simulink model "BLEMeshPDRvsRateModel"  (R2021a)
settings: Solver=VariableStepDiscrete  StartTime=0.0  StopTime=5  MaxStep=inf  RelTol=1e-3
PostLoadFcn:
  | load('bleMeshBusObjects.mat');
  | load('bleMeshDESNodePositions.mat');
  | ModelName = bdroot;
  | helperBLEMeshAssignNodeIDs(ModelName);
  | NumberOfNodes = numel(helperBLEMeshGetNodeNamesList(ModelName));
  | % Statistics
  | opcode = 0; % For creating the table
  | helperBLEMeshUpdateStatistics(opcode);
  | meshNetworkGraph = helperBLEMeshVisualizeNetwork();
InitFcn:
  | load('bleMeshBusObjects.mat');
  | load('bleMeshDESNodePositions.mat');
  | ModelName = bdroot;
  | helperBLEMeshAssignNodeIDs(ModelName);
  | NumberOfNodes = numel(helperBLEMeshGetNodeNamesList(ModelName));
  | % Statistics
  | opcode = 0; % For creating the table
  | helperBLEMeshUpdateStatistics(opcode);
  | meshNetworkGraph = helperBLEMeshVisualizeNetwork();
  | rng('default');
StartFcn:
  | if enableVisualization == 1
  | meshNetworkGraph.createNetwork();
  | end
StopFcn:
  | % Sort statisticsAtEachNode table
  | list = statisticsAtEachNode.Properties.RowNames;
  | nodeNum = cellfun(@(x)sscanf(x,'Node%d'), list);
  | [~,sortIdx] = sort(nodeNum);
  | statisticsAtEachNode = statisticsAtEachNode(sortIdx, :);
  | 
  | % Fill node statisticsAtEachNode in a cell array as input to visualization object
  | nodeStatistics = cell(1, NumberOfNodes);
  | for idx = 1:NumberOfNodes
  |     stats = {
  |         'Node Type', statisticsAtEachNode{idx, 'NodeType'}, ...
  |         'PHYTransmittedSignals', statisticsAtEachNode{idx, 'PHYTransmittedSignals'}, ...
  |         'PHYReceivedSignals', statisticsAtEachNode{idx, 'PHYReceivedSignals'}, ...
  |         'TotalCollisions', statisticsAtEachNode{idx, 'TotalCollisions'}, ...
  |         'LinkLayerTransmittedMsgs', statisticsAtEachNode{idx, 'LinkLayerTransmittedMsgs'}, ...
  |         'LinkLayerReceivedMsgs', statisticsAtEachNode{idx, 'LinkLayerReceivedMsgs'}, ...
  |         'CRCFailedMsgs', statisticsAtEachNode{idx, 'CRCFailedMsgs'}, ...
  |         'NetworkLayerTransmittedMsgs', statisticsAtEachNode{idx, 'NetworkLayerTransmittedMsgs'}, ...
  |         'NetworkLayerReceivedMsgs', statisticsAtEachNode{idx, 'NetworkLayerReceivedMsgs'}, ...
  |         'ReceivedApplicationMsgs', statisticsAtEachNode{idx, 'ReceivedApplicationMsgs'}, ...
  |         'NetworkLayerRelayedMsgs', statisticsAtEachNode{idx, 'NetworkLayerRelayedMsgs'}, ...
  |         'NetworkLayerDroppedMsgs', statisticsAtEachNode{idx, 'NetworkLayerDroppedMsgs'}};
  |     nodeStatistics{idx} = stats;
  | end
  | % Update statisticsAtEachNode in visualization object
  | if enableVisualization == 1
  | meshNetworkGraph.updateNodeStatistics(nodeStatistics);
  | end
  | % Calculate PDR of network
  | PDR = sum(statisticsAtEachNode.ReceivedApplicationMsgs) / sum(statisticsAtEachNode.NetworkLayerTransmittedMsgs);
  | fprintf('Network PDR is: %f\n', round(PDR, 4));
values from neighbouring files (symbols this model uses):
  bleMeshDESNodePositions = [0 2 4 6 8 10 12 14 16 18 20 22 ... (300 elements, 100x3)]    [bleMeshDESNodePositions.mat]    (also in bleMeshDESNodePositions19.mat = [5.030833333 8.024583333 13.395 16.32708333 22.90125 22.9012; bleMeshDESNodePositions38.mat = [2.7 5.45 5.825 10.65 13.5 13.875 18.65 21.4 18.55 2.7 5.45 ; bleMeshDESNodePositions51.mat = [2.45 5.4 2.45 5.4 5.75 10.375 13.3 10.375 13.3 13.75 18.75 ; bleMeshDESNodePositions68.mat = [0 2 4 6 8 10 12 14 16 18 0 2 ... (300 elements, 100x3)])
undefined symbols (not defined in the file or in its folder): m
libraries: BLEMeshLib x260
(part 2 of 5)

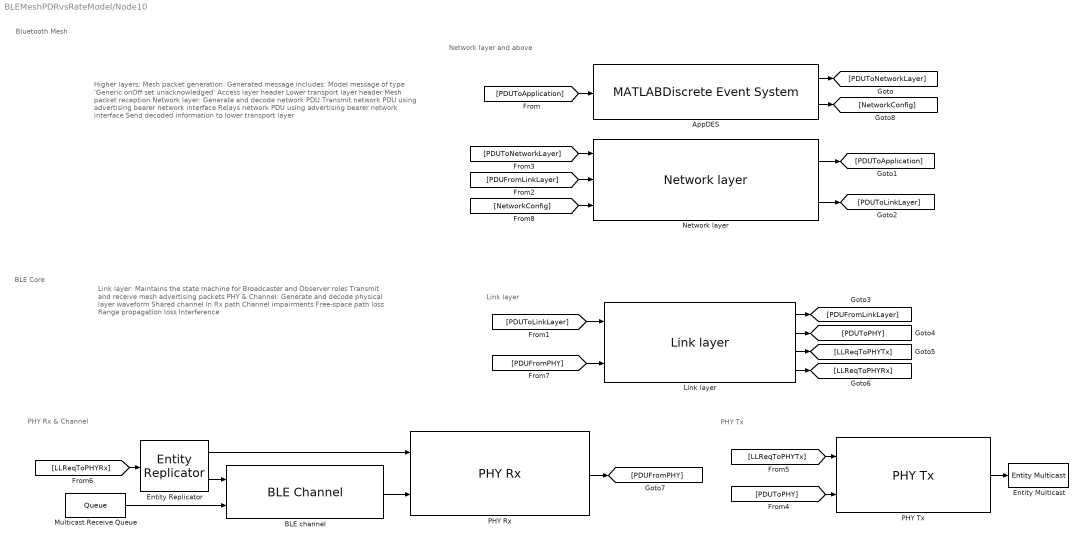
== system BLEMeshPDRvsRateModel/Node10 ==
  note: Network layer and above
  note: Link layer
  note: Link layer:
      | Maintains the state machine for Broadcaster and Observer roles
      | Transmit and receive mesh advertising packets
      |
      | PHY & Channel:
      | Generate and decode physical layer waveform
      | Shared channel in Rx path
      | Channel impairments
      | Free-space path loss
      | Range propagation loss
      | Interference
  note: BLE Core
  note: Bluetooth Mesh
  note: PHY Rx & Channel
  note: PHY Tx
  note: Higher layers:
      | Mesh packet generation. Generated message includes:
      | Model message of type 'Generic onOff set unacknowledged'
      | Access layer header
      | Lower transport layer header
      | Mesh packet reception
      |
      | Network layer:
      | Generate and decode network PDU
      | Transmit network PDU using advertising bearer network interface
      | Relays network PDU using advertising bearer network interface
      | Send decoded information to lower transport layer
  AppDES : MATLABDiscreteEventSystem  InputPortMessageModes=m  OutputPortMessageModes=m,m  System=AppDES  NodeID=1  DestinationNode=1  ApplicationState=0  TTL=127  SourceRate=1  TotalPackets=1  SimulateUsing=Code generation
      mask Type: AppDES
      mask Display:
      | disp('AppDES');
      | port_label('input',1,'transportPDUIn');
      | port_label('output',1,'transportPDUOut');
      | port_label('output',2,'networkConfig');
  BLE channel : BLEMeshLib/BLE Channel  RangePropagationLoss=On  FSPLModel=On  RxRange=8  NodePosition=NodePosition  NodeID=NodeID  SimulateUsing=Code generation
  Entity Multicast : EntityMulticast  InputPortMessageModes=m  MulticastTag=channel
  Entity Replicator : EntityReplicator  InputPortMessageModes=m  OutputPortMessageModes=m,m
  Link layer : BLEMeshLib/Link layer  RandomAdvertising=On  AdvertisingInterval=20  ScanInterval=30  NodeID=NodeID  SimulateUsing=Code generation  mask(helperBLEMeshLinkLayerDES){}
  Multicast Receive Queue : Queue  OutputPortMessageModes=m  EntityArrivalSource=Multicast  MulticastTag=channel
  Network layer : BLEMeshLib/Network layer  Relay=Off  ElementAddresses=ElementAddress  NetworkTransmitCount=3  NetworkTransmitInterval=30  RelayRetransmitCount=3  RelayRetransmitInterval=30  NodeID=NodeID  SimulateUsing=Code generation
  PHY Rx : BLEMeshLib/PHY Rx  NoiseFigure=0  NodeID=NodeID  SimulateUsing=Interpreted execution
  PHY Tx : BLEMeshLib/PHY Tx  TxPower=0  NodePosition=NodePosition  NodeID=NodeID  SimulateUsing=Interpreted execution
  wires:
  Link layer/4 -> [LLReqToPHYRx]
  Link layer/2 -> [PDUToPHY]
  Link layer/3 -> [LLReqToPHYTx]
  Link layer/1 -> [PDUFromLinkLayer]
  [PDUToNetworkLayer] -> Network layer/1
  Network layer/1 -> [PDUToApplication]
  [PDUFromLinkLayer] -> Network layer/2
  Entity Replicator/1 -> PHY Rx/1
  PHY Rx/1 -> [PDUFromPHY]
  BLE channel/1 -> PHY Rx/2
  PHY Tx/1 -> Entity Multicast/1
  [LLReqToPHYRx] -> Entity Replicator/1
  Multicast Receive Queue/1 -> BLE channel/2
  Entity Replicator/2 -> BLE channel/1
  [LLReqToPHYTx] -> PHY Tx/1
  [PDUToPHY] -> PHY Tx/2
  Network layer/2 -> [PDUToLinkLayer]
  [PDUToLinkLayer] -> Link layer/1
  [PDUFromPHY] -> Link layer/2
  AppDES/1 -> [PDUToNetworkLayer]
  [PDUToApplication] -> AppDES/1
  [NetworkConfig] -> Network layer/3
  AppDES/2 -> [NetworkConfig]

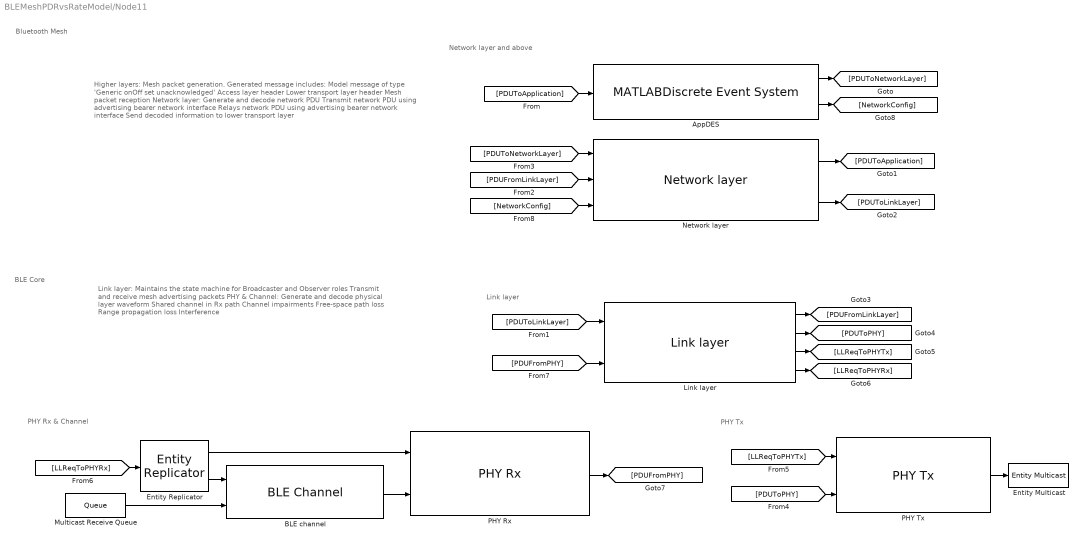
== system BLEMeshPDRvsRateModel/Node11 ==
  note: Network layer and above
  note: Link layer
  note: Link layer:
      | Maintains the state machine for Broadcaster and Observer roles
      | Transmit and receive mesh advertising packets
      |
      | PHY & Channel:
      | Generate and decode physical layer waveform
      | Shared channel in Rx path
      | Channel impairments
      | Free-space path loss
      | Range propagation loss
      | Interference
  note: BLE Core
  note: Bluetooth Mesh
  note: PHY Rx & Channel
  note: PHY Tx
  note: Higher layers:
      | Mesh packet generation. Generated message includes:
      | Model message of type 'Generic onOff set unacknowledged'
      | Access layer header
      | Lower transport layer header
      | Mesh packet reception
      |
      | Network layer:
      | Generate and decode network PDU
      | Transmit network PDU using advertising bearer network interface
      | Relays network PDU using advertising bearer network interface
      | Send decoded information to lower transport layer
  AppDES : MATLABDiscreteEventSystem  InputPortMessageModes=m  OutputPortMessageModes=m,m  System=AppDES  NodeID=1  DestinationNode=1  ApplicationState=0  TTL=127  SourceRate=1  TotalPackets=1  SimulateUsing=Code generation
      mask Type: AppDES
      mask Display:
      | disp('AppDES');
      | port_label('input',1,'transportPDUIn');
      | port_label('output',1,'transportPDUOut');
      | port_label('output',2,'networkConfig');
  BLE channel : BLEMeshLib/BLE Channel  RangePropagationLoss=On  FSPLModel=On  RxRange=8  NodePosition=NodePosition  NodeID=NodeID  SimulateUsing=Code generation
  Entity Multicast : EntityMulticast  InputPortMessageModes=m  MulticastTag=channel
  Entity Replicator : EntityReplicator  InputPortMessageModes=m  OutputPortMessageModes=m,m
  Link layer : BLEMeshLib/Link layer  RandomAdvertising=On  AdvertisingInterval=20  ScanInterval=30  NodeID=NodeID  SimulateUsing=Code generation  mask(helperBLEMeshLinkLayerDES){}
  Multicast Receive Queue : Queue  OutputPortMessageModes=m  EntityArrivalSource=Multicast  MulticastTag=channel
  Network layer : BLEMeshLib/Network layer  Relay=On  ElementAddresses=ElementAddress  NetworkTransmitCount=3  NetworkTransmitInterval=30  RelayRetransmitCount=3  RelayRetransmitInterval=30  NodeID=NodeID  SimulateUsing=Code generation
  PHY Rx : BLEMeshLib/PHY Rx  NoiseFigure=0  NodeID=NodeID  SimulateUsing=Interpreted execution
  PHY Tx : BLEMeshLib/PHY Tx  TxPower=0  NodePosition=NodePosition  NodeID=NodeID  SimulateUsing=Interpreted execution
  wires:
  Link layer/4 -> [LLReqToPHYRx]
  Link layer/2 -> [PDUToPHY]
  Link layer/3 -> [LLReqToPHYTx]
  Link layer/1 -> [PDUFromLinkLayer]
  [PDUToNetworkLayer] -> Network layer/1
  Network layer/1 -> [PDUToApplication]
  [PDUFromLinkLayer] -> Network layer/2
  Entity Replicator/1 -> PHY Rx/1
  PHY Rx/1 -> [PDUFromPHY]
  BLE channel/1 -> PHY Rx/2
  PHY Tx/1 -> Entity Multicast/1
  [LLReqToPHYRx] -> Entity Replicator/1
  Multicast Receive Queue/1 -> BLE channel/2
  Entity Replicator/2 -> BLE channel/1
  [LLReqToPHYTx] -> PHY Tx/1
  [PDUToPHY] -> PHY Tx/2
  Network layer/2 -> [PDUToLinkLayer]
  [PDUToLinkLayer] -> Link layer/1
  [PDUFromPHY] -> Link layer/2
  AppDES/1 -> [PDUToNetworkLayer]
  [PDUToApplication] -> AppDES/1
  [NetworkConfig] -> Network layer/3
  AppDES/2 -> [NetworkConfig]

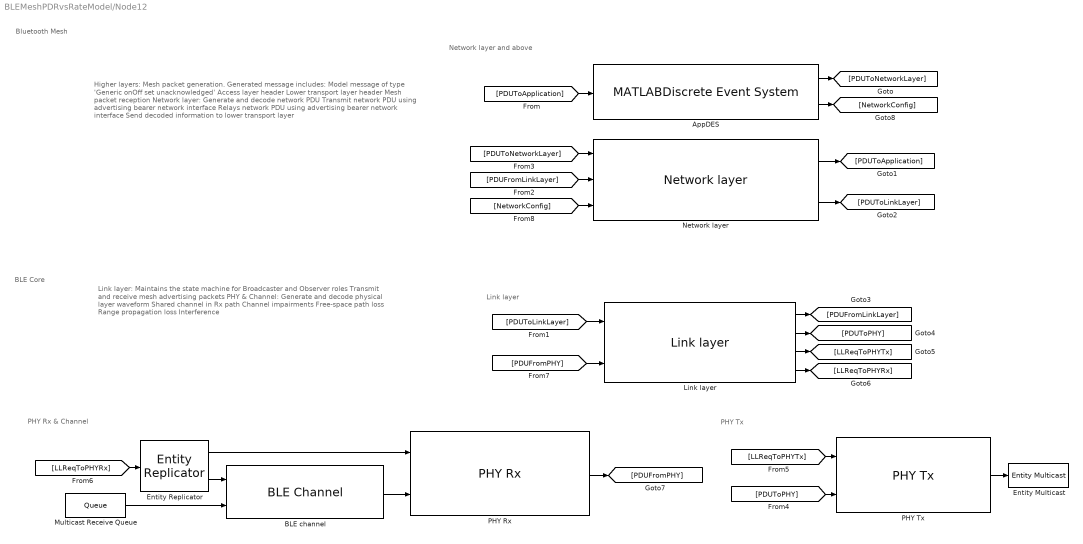
== system BLEMeshPDRvsRateModel/Node12 ==
  note: Network layer and above
  note: Link layer
  note: Link layer:
      | Maintains the state machine for Broadcaster and Observer roles
      | Transmit and receive mesh advertising packets
      |
      | PHY & Channel:
      | Generate and decode physical layer waveform
      | Shared channel in Rx path
      | Channel impairments
      | Free-space path loss
      | Range propagation loss
      | Interference
  note: BLE Core
  note: Bluetooth Mesh
  note: PHY Rx & Channel
  note: PHY Tx
  note: Higher layers:
      | Mesh packet generation. Generated message includes:
      | Model message of type 'Generic onOff set unacknowledged'
      | Access layer header
      | Lower transport layer header
      | Mesh packet reception
      |
      | Network layer:
      | Generate and decode network PDU
      | Transmit network PDU using advertising bearer network interface
      | Relays network PDU using advertising bearer network interface
      | Send decoded information to lower transport layer
  AppDES : MATLABDiscreteEventSystem  InputPortMessageModes=m  OutputPortMessageModes=m,m  System=AppDES  NodeID=1  DestinationNode=1  ApplicationState=0  TTL=127  SourceRate=1  TotalPackets=1  SimulateUsing=Code generation
      mask Type: AppDES
      mask Display:
      | disp('AppDES');
      | port_label('input',1,'transportPDUIn');
      | port_label('output',1,'transportPDUOut');
      | port_label('output',2,'networkConfig');
  BLE channel : BLEMeshLib/BLE Channel  RangePropagationLoss=On  FSPLModel=On  RxRange=8  NodePosition=NodePosition  NodeID=NodeID  SimulateUsing=Code generation
  Entity Multicast : EntityMulticast  InputPortMessageModes=m  MulticastTag=channel
  Entity Replicator : EntityReplicator  InputPortMessageModes=m  OutputPortMessageModes=m,m
  Link layer : BLEMeshLib/Link layer  RandomAdvertising=On  AdvertisingInterval=20  ScanInterval=30  NodeID=NodeID  SimulateUsing=Code generation  mask(helperBLEMeshLinkLayerDES){}
  Multicast Receive Queue : Queue  OutputPortMessageModes=m  EntityArrivalSource=Multicast  MulticastTag=channel
  Network layer : BLEMeshLib/Network layer  Relay=On  ElementAddresses=ElementAddress  NetworkTransmitCount=3  NetworkTransmitInterval=30  RelayRetransmitCount=3  RelayRetransmitInterval=30  NodeID=NodeID  SimulateUsing=Code generation
  PHY Rx : BLEMeshLib/PHY Rx  NoiseFigure=0  NodeID=NodeID  SimulateUsing=Interpreted execution
  PHY Tx : BLEMeshLib/PHY Tx  TxPower=0  NodePosition=NodePosition  NodeID=NodeID  SimulateUsing=Interpreted execution
  wires:
  Link layer/4 -> [LLReqToPHYRx]
  Link layer/2 -> [PDUToPHY]
  Link layer/3 -> [LLReqToPHYTx]
  Link layer/1 -> [PDUFromLinkLayer]
  [PDUToNetworkLayer] -> Network layer/1
  Network layer/1 -> [PDUToApplication]
  [PDUFromLinkLayer] -> Network layer/2
  Entity Replicator/1 -> PHY Rx/1
  PHY Rx/1 -> [PDUFromPHY]
  BLE channel/1 -> PHY Rx/2
  PHY Tx/1 -> Entity Multicast/1
  [LLReqToPHYRx] -> Entity Replicator/1
  Multicast Receive Queue/1 -> BLE channel/2
  Entity Replicator/2 -> BLE channel/1
  [LLReqToPHYTx] -> PHY Tx/1
  [PDUToPHY] -> PHY Tx/2
  Network layer/2 -> [PDUToLinkLayer]
  [PDUToLinkLayer] -> Link layer/1
  [PDUFromPHY] -> Link layer/2
  AppDES/1 -> [PDUToNetworkLayer]
  [PDUToApplication] -> AppDES/1
  [NetworkConfig] -> Network layer/3
  AppDES/2 -> [NetworkConfig]

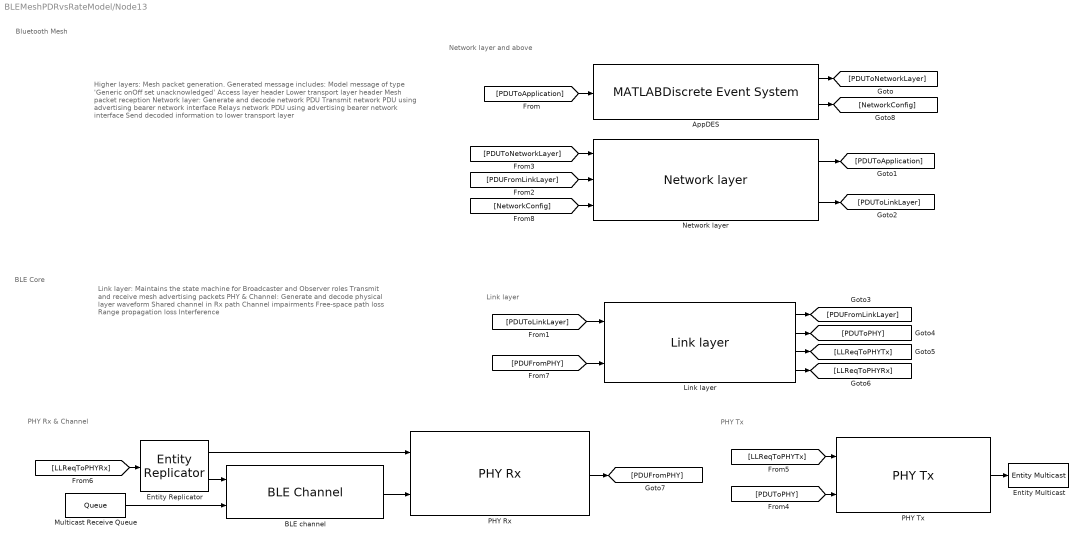
== system BLEMeshPDRvsRateModel/Node13 ==
  note: Network layer and above
  note: Link layer
  note: Link layer:
      | Maintains the state machine for Broadcaster and Observer roles
      | Transmit and receive mesh advertising packets
      |
      | PHY & Channel:
      | Generate and decode physical layer waveform
      | Shared channel in Rx path
      | Channel impairments
      | Free-space path loss
      | Range propagation loss
      | Interference
  note: BLE Core
  note: Bluetooth Mesh
  note: PHY Rx & Channel
  note: PHY Tx
  note: Higher layers:
      | Mesh packet generation. Generated message includes:
      | Model message of type 'Generic onOff set unacknowledged'
      | Access layer header
      | Lower transport layer header
      | Mesh packet reception
      |
      | Network layer:
      | Generate and decode network PDU
      | Transmit network PDU using advertising bearer network interface
      | Relays network PDU using advertising bearer network interface
      | Send decoded information to lower transport layer
  AppDES : MATLABDiscreteEventSystem  InputPortMessageModes=m  OutputPortMessageModes=m,m  System=AppDES  NodeID=1  DestinationNode=1  ApplicationState=0  TTL=127  SourceRate=1  TotalPackets=1  SimulateUsing=Code generation
      mask Type: AppDES
      mask Display:
      | disp('AppDES');
      | port_label('input',1,'transportPDUIn');
      | port_label('output',1,'transportPDUOut');
      | port_label('output',2,'networkConfig');
  BLE channel : BLEMeshLib/BLE Channel  RangePropagationLoss=On  FSPLModel=On  RxRange=8  NodePosition=NodePosition  NodeID=NodeID  SimulateUsing=Code generation
  Entity Multicast : EntityMulticast  InputPortMessageModes=m  MulticastTag=channel
  Entity Replicator : EntityReplicator  InputPortMessageModes=m  OutputPortMessageModes=m,m
  Link layer : BLEMeshLib/Link layer  RandomAdvertising=On  AdvertisingInterval=20  ScanInterval=30  NodeID=NodeID  SimulateUsing=Code generation  mask(helperBLEMeshLinkLayerDES){}
  Multicast Receive Queue : Queue  OutputPortMessageModes=m  EntityArrivalSource=Multicast  MulticastTag=channel
  Network layer : BLEMeshLib/Network layer  Relay=On  ElementAddresses=ElementAddress  NetworkTransmitCount=3  NetworkTransmitInterval=30  RelayRetransmitCount=3  RelayRetransmitInterval=30  NodeID=NodeID  SimulateUsing=Code generation
  PHY Rx : BLEMeshLib/PHY Rx  NoiseFigure=0  NodeID=NodeID  SimulateUsing=Interpreted execution
  PHY Tx : BLEMeshLib/PHY Tx  TxPower=0  NodePosition=NodePosition  NodeID=NodeID  SimulateUsing=Interpreted execution
  wires:
  Link layer/4 -> [LLReqToPHYRx]
  Link layer/2 -> [PDUToPHY]
  Link layer/3 -> [LLReqToPHYTx]
  Link layer/1 -> [PDUFromLinkLayer]
  [PDUToNetworkLayer] -> Network layer/1
  Network layer/1 -> [PDUToApplication]
  [PDUFromLinkLayer] -> Network layer/2
  Entity Replicator/1 -> PHY Rx/1
  PHY Rx/1 -> [PDUFromPHY]
  BLE channel/1 -> PHY Rx/2
  PHY Tx/1 -> Entity Multicast/1
  [LLReqToPHYRx] -> Entity Replicator/1
  Multicast Receive Queue/1 -> BLE channel/2
  Entity Replicator/2 -> BLE channel/1
  [LLReqToPHYTx] -> PHY Tx/1
  [PDUToPHY] -> PHY Tx/2
  Network layer/2 -> [PDUToLinkLayer]
  [PDUToLinkLayer] -> Link layer/1
  [PDUFromPHY] -> Link layer/2
  AppDES/1 -> [PDUToNetworkLayer]
  [PDUToApplication] -> AppDES/1
  [NetworkConfig] -> Network layer/3
  AppDES/2 -> [NetworkConfig]

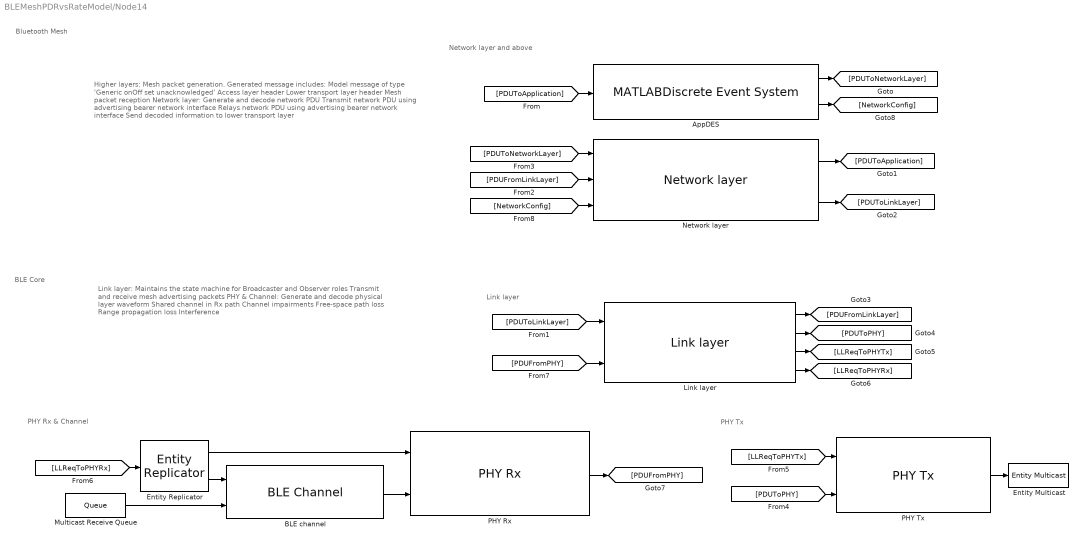
== system BLEMeshPDRvsRateModel/Node14 ==
  note: Network layer and above
  note: Link layer
  note: Link layer:
      | Maintains the state machine for Broadcaster and Observer roles
      | Transmit and receive mesh advertising packets
      |
      | PHY & Channel:
      | Generate and decode physical layer waveform
      | Shared channel in Rx path
      | Channel impairments
      | Free-space path loss
      | Range propagation loss
      | Interference
  note: BLE Core
  note: Bluetooth Mesh
  note: PHY Rx & Channel
  note: PHY Tx
  note: Higher layers:
      | Mesh packet generation. Generated message includes:
      | Model message of type 'Generic onOff set unacknowledged'
      | Access layer header
      | Lower transport layer header
      | Mesh packet reception
      |
      | Network layer:
      | Generate and decode network PDU
      | Transmit network PDU using advertising bearer network interface
      | Relays network PDU using advertising bearer network interface
      | Send decoded information to lower transport layer
  AppDES : MATLABDiscreteEventSystem  InputPortMessageModes=m  OutputPortMessageModes=m,m  System=AppDES  NodeID=1  DestinationNode=1  ApplicationState=0  TTL=127  SourceRate=1  TotalPackets=1  SimulateUsing=Code generation
      mask Type: AppDES
      mask Display:
      | disp('AppDES');
      | port_label('input',1,'transportPDUIn');
      | port_label('output',1,'transportPDUOut');
      | port_label('output',2,'networkConfig');
  BLE channel : BLEMeshLib/BLE Channel  RangePropagationLoss=On  FSPLModel=On  RxRange=8  NodePosition=NodePosition  NodeID=NodeID  SimulateUsing=Code generation
  Entity Multicast : EntityMulticast  InputPortMessageModes=m  MulticastTag=channel
  Entity Replicator : EntityReplicator  InputPortMessageModes=m  OutputPortMessageModes=m,m
  Link layer : BLEMeshLib/Link layer  RandomAdvertising=On  AdvertisingInterval=20  ScanInterval=30  NodeID=NodeID  SimulateUsing=Code generation  mask(helperBLEMeshLinkLayerDES){}
  Multicast Receive Queue : Queue  OutputPortMessageModes=m  EntityArrivalSource=Multicast  MulticastTag=channel
  Network layer : BLEMeshLib/Network layer  Relay=On  ElementAddresses=ElementAddress  NetworkTransmitCount=3  NetworkTransmitInterval=30  RelayRetransmitCount=3  RelayRetransmitInterval=30  NodeID=NodeID  SimulateUsing=Code generation
  PHY Rx : BLEMeshLib/PHY Rx  NoiseFigure=0  NodeID=NodeID  SimulateUsing=Interpreted execution
  PHY Tx : BLEMeshLib/PHY Tx  TxPower=0  NodePosition=NodePosition  NodeID=NodeID  SimulateUsing=Interpreted execution
  wires:
  Link layer/4 -> [LLReqToPHYRx]
  Link layer/2 -> [PDUToPHY]
  Link layer/3 -> [LLReqToPHYTx]
  Link layer/1 -> [PDUFromLinkLayer]
  [PDUToNetworkLayer] -> Network layer/1
  Network layer/1 -> [PDUToApplication]
  [PDUFromLinkLayer] -> Network layer/2
  Entity Replicator/1 -> PHY Rx/1
  PHY Rx/1 -> [PDUFromPHY]
  BLE channel/1 -> PHY Rx/2
  PHY Tx/1 -> Entity Multicast/1
  [LLReqToPHYRx] -> Entity Replicator/1
  Multicast Receive Queue/1 -> BLE channel/2
  Entity Replicator/2 -> BLE channel/1
  [LLReqToPHYTx] -> PHY Tx/1
  [PDUToPHY] -> PHY Tx/2
  Network layer/2 -> [PDUToLinkLayer]
  [PDUToLinkLayer] -> Link layer/1
  [PDUFromPHY] -> Link layer/2
  AppDES/1 -> [PDUToNetworkLayer]
  [PDUToApplication] -> AppDES/1
  [NetworkConfig] -> Network layer/3
  AppDES/2 -> [NetworkConfig]

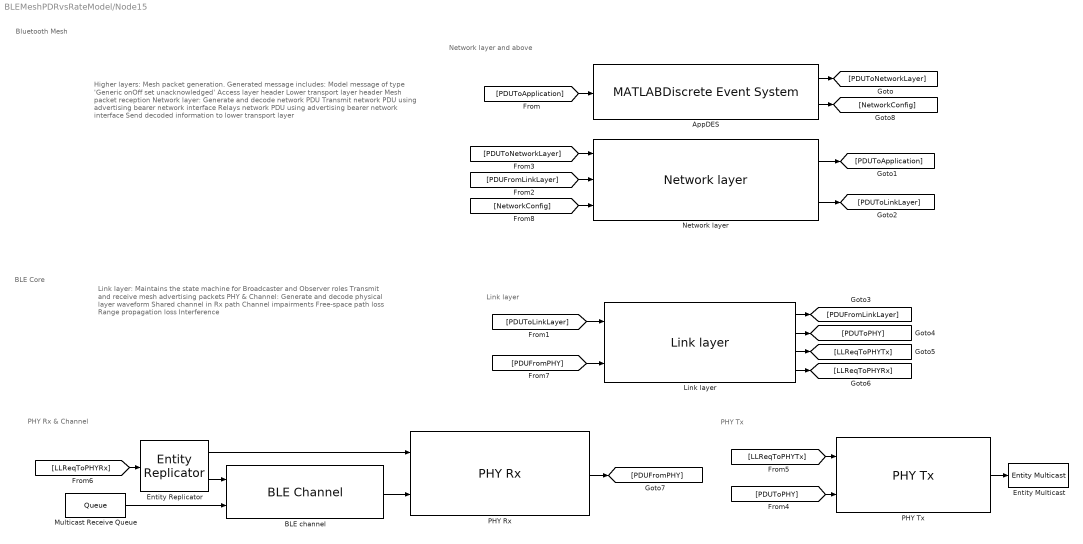
== system BLEMeshPDRvsRateModel/Node15 ==
  note: Network layer and above
  note: Link layer
  note: Link layer:
      | Maintains the state machine for Broadcaster and Observer roles
      | Transmit and receive mesh advertising packets
      |
      | PHY & Channel:
      | Generate and decode physical layer waveform
      | Shared channel in Rx path
      | Channel impairments
      | Free-space path loss
      | Range propagation loss
      | Interference
  note: BLE Core
  note: Bluetooth Mesh
  note: PHY Rx & Channel
  note: PHY Tx
  note: Higher layers:
      | Mesh packet generation. Generated message includes:
      | Model message of type 'Generic onOff set unacknowledged'
      | Access layer header
      | Lower transport layer header
      | Mesh packet reception
      |
      | Network layer:
      | Generate and decode network PDU
      | Transmit network PDU using advertising bearer network interface
      | Relays network PDU using advertising bearer network interface
      | Send decoded information to lower transport layer
  AppDES : MATLABDiscreteEventSystem  InputPortMessageModes=m  OutputPortMessageModes=m,m  System=AppDES  NodeID=1  DestinationNode=1  ApplicationState=0  TTL=127  SourceRate=1  TotalPackets=1  SimulateUsing=Code generation
      mask Type: AppDES
      mask Display:
      | disp('AppDES');
      | port_label('input',1,'transportPDUIn');
      | port_label('output',1,'transportPDUOut');
      | port_label('output',2,'networkConfig');
  BLE channel : BLEMeshLib/BLE Channel  RangePropagationLoss=On  FSPLModel=On  RxRange=8  NodePosition=NodePosition  NodeID=NodeID  SimulateUsing=Code generation
  Entity Multicast : EntityMulticast  InputPortMessageModes=m  MulticastTag=channel
  Entity Replicator : EntityReplicator  InputPortMessageModes=m  OutputPortMessageModes=m,m
  Link layer : BLEMeshLib/Link layer  RandomAdvertising=On  AdvertisingInterval=20  ScanInterval=30  NodeID=NodeID  SimulateUsing=Code generation  mask(helperBLEMeshLinkLayerDES){}
  Multicast Receive Queue : Queue  OutputPortMessageModes=m  EntityArrivalSource=Multicast  MulticastTag=channel
  Network layer : BLEMeshLib/Network layer  Relay=Off  ElementAddresses=ElementAddress  NetworkTransmitCount=3  NetworkTransmitInterval=30  RelayRetransmitCount=3  RelayRetransmitInterval=30  NodeID=NodeID  SimulateUsing=Code generation
  PHY Rx : BLEMeshLib/PHY Rx  NoiseFigure=0  NodeID=NodeID  SimulateUsing=Interpreted execution
  PHY Tx : BLEMeshLib/PHY Tx  TxPower=0  NodePosition=NodePosition  NodeID=NodeID  SimulateUsing=Interpreted execution
  wires:
  Link layer/4 -> [LLReqToPHYRx]
  Link layer/2 -> [PDUToPHY]
  Link layer/3 -> [LLReqToPHYTx]
  Link layer/1 -> [PDUFromLinkLayer]
  [PDUToNetworkLayer] -> Network layer/1
  Network layer/1 -> [PDUToApplication]
  [PDUFromLinkLayer] -> Network layer/2
  Entity Replicator/1 -> PHY Rx/1
  PHY Rx/1 -> [PDUFromPHY]
  BLE channel/1 -> PHY Rx/2
  PHY Tx/1 -> Entity Multicast/1
  [LLReqToPHYRx] -> Entity Replicator/1
  Multicast Receive Queue/1 -> BLE channel/2
  Entity Replicator/2 -> BLE channel/1
  [LLReqToPHYTx] -> PHY Tx/1
  [PDUToPHY] -> PHY Tx/2
  Network layer/2 -> [PDUToLinkLayer]
  [PDUToLinkLayer] -> Link layer/1
  [PDUFromPHY] -> Link layer/2
  AppDES/1 -> [PDUToNetworkLayer]
  [PDUToApplication] -> AppDES/1
  [NetworkConfig] -> Network layer/3
  AppDES/2 -> [NetworkConfig]

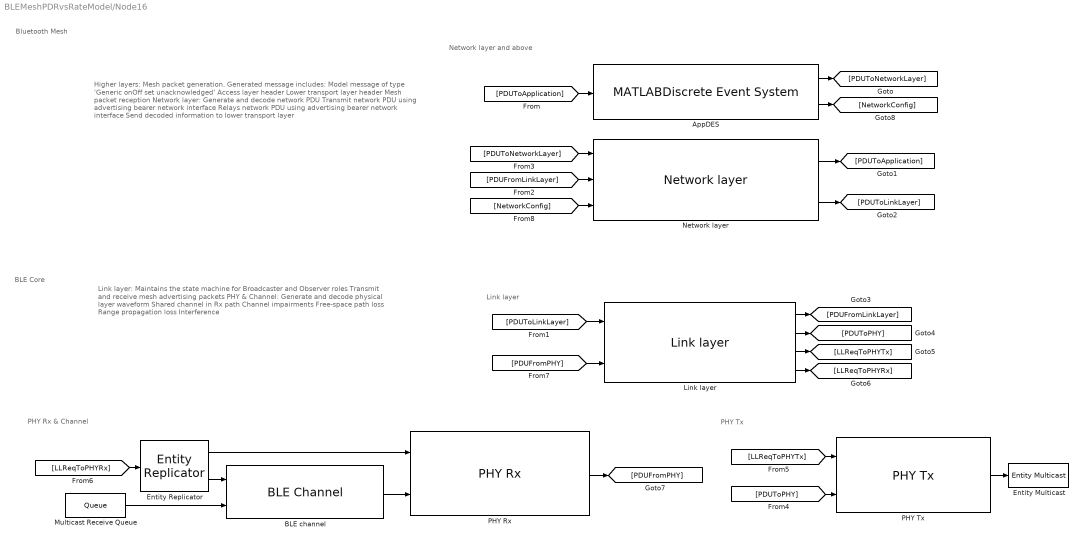
== system BLEMeshPDRvsRateModel/Node16 ==
  note: Network layer and above
  note: Link layer
  note: Link layer:
      | Maintains the state machine for Broadcaster and Observer roles
      | Transmit and receive mesh advertising packets
      |
      | PHY & Channel:
      | Generate and decode physical layer waveform
      | Shared channel in Rx path
      | Channel impairments
      | Free-space path loss
      | Range propagation loss
      | Interference
  note: BLE Core
  note: Bluetooth Mesh
  note: PHY Rx & Channel
  note: PHY Tx
  note: Higher layers:
      | Mesh packet generation. Generated message includes:
      | Model message of type 'Generic onOff set unacknowledged'
      | Access layer header
      | Lower transport layer header
      | Mesh packet reception
      |
      | Network layer:
      | Generate and decode network PDU
      | Transmit network PDU using advertising bearer network interface
      | Relays network PDU using advertising bearer network interface
      | Send decoded information to lower transport layer
  AppDES : MATLABDiscreteEventSystem  InputPortMessageModes=m  OutputPortMessageModes=m,m  System=AppDES  NodeID=1  DestinationNode=1  ApplicationState=0  TTL=127  SourceRate=1  TotalPackets=1  SimulateUsing=Code generation
      mask Type: AppDES
      mask Display:
      | disp('AppDES');
      | port_label('input',1,'transportPDUIn');
      | port_label('output',1,'transportPDUOut');
      | port_label('output',2,'networkConfig');
  BLE channel : BLEMeshLib/BLE Channel  RangePropagationLoss=On  FSPLModel=On  RxRange=8  NodePosition=NodePosition  NodeID=NodeID  SimulateUsing=Code generation
  Entity Multicast : EntityMulticast  InputPortMessageModes=m  MulticastTag=channel
  Entity Replicator : EntityReplicator  InputPortMessageModes=m  OutputPortMessageModes=m,m
  Link layer : BLEMeshLib/Link layer  RandomAdvertising=On  AdvertisingInterval=20  ScanInterval=30  NodeID=NodeID  SimulateUsing=Code generation  mask(helperBLEMeshLinkLayerDES){}
  Multicast Receive Queue : Queue  OutputPortMessageModes=m  EntityArrivalSource=Multicast  MulticastTag=channel
  Network layer : BLEMeshLib/Network layer  Relay=Off  ElementAddresses=ElementAddress  NetworkTransmitCount=3  NetworkTransmitInterval=30  RelayRetransmitCount=3  RelayRetransmitInterval=30  NodeID=NodeID  SimulateUsing=Code generation
  PHY Rx : BLEMeshLib/PHY Rx  NoiseFigure=0  NodeID=NodeID  SimulateUsing=Interpreted execution
  PHY Tx : BLEMeshLib/PHY Tx  TxPower=0  NodePosition=NodePosition  NodeID=NodeID  SimulateUsing=Interpreted execution
  wires:
  Link layer/4 -> [LLReqToPHYRx]
  Link layer/2 -> [PDUToPHY]
  Link layer/3 -> [LLReqToPHYTx]
  Link layer/1 -> [PDUFromLinkLayer]
  [PDUToNetworkLayer] -> Network layer/1
  Network layer/1 -> [PDUToApplication]
  [PDUFromLinkLayer] -> Network layer/2
  Entity Replicator/1 -> PHY Rx/1
  PHY Rx/1 -> [PDUFromPHY]
  BLE channel/1 -> PHY Rx/2
  PHY Tx/1 -> Entity Multicast/1
  [LLReqToPHYRx] -> Entity Replicator/1
  Multicast Receive Queue/1 -> BLE channel/2
  Entity Replicator/2 -> BLE channel/1
  [LLReqToPHYTx] -> PHY Tx/1
  [PDUToPHY] -> PHY Tx/2
  Network layer/2 -> [PDUToLinkLayer]
  [PDUToLinkLayer] -> Link layer/1
  [PDUFromPHY] -> Link layer/2
  AppDES/1 -> [PDUToNetworkLayer]
  [PDUToApplication] -> AppDES/1
  [NetworkConfig] -> Network layer/3
  AppDES/2 -> [NetworkConfig]

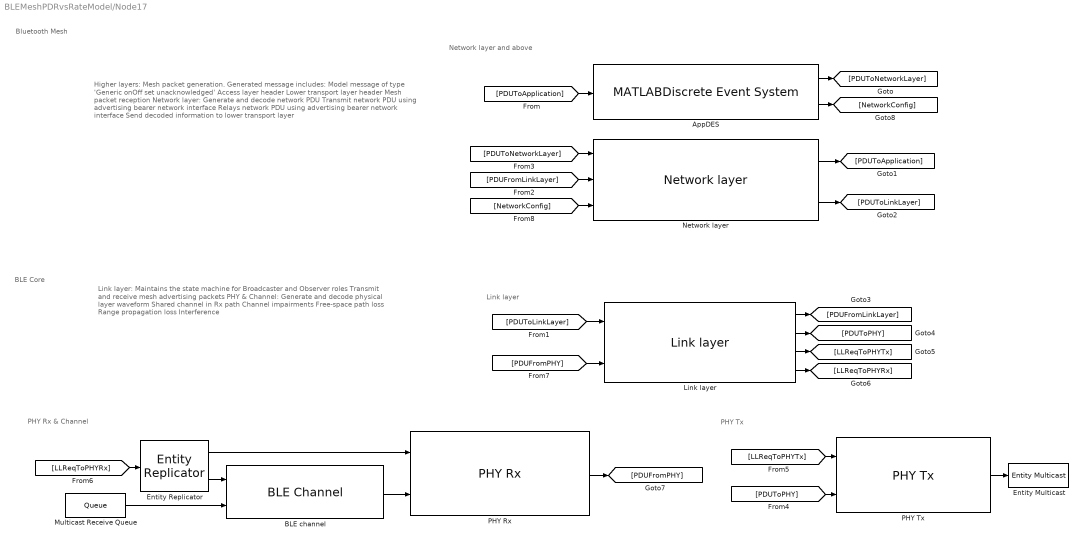
== system BLEMeshPDRvsRateModel/Node17 ==
  note: Network layer and above
  note: Link layer
  note: Link layer:
      | Maintains the state machine for Broadcaster and Observer roles
      | Transmit and receive mesh advertising packets
      |
      | PHY & Channel:
      | Generate and decode physical layer waveform
      | Shared channel in Rx path
      | Channel impairments
      | Free-space path loss
      | Range propagation loss
      | Interference
  note: BLE Core
  note: Bluetooth Mesh
  note: PHY Rx & Channel
  note: PHY Tx
  note: Higher layers:
      | Mesh packet generation. Generated message includes:
      | Model message of type 'Generic onOff set unacknowledged'
      | Access layer header
      | Lower transport layer header
      | Mesh packet reception
      |
      | Network layer:
      | Generate and decode network PDU
      | Transmit network PDU using advertising bearer network interface
      | Relays network PDU using advertising bearer network interface
      | Send decoded information to lower transport layer
  AppDES : MATLABDiscreteEventSystem  InputPortMessageModes=m  OutputPortMessageModes=m,m  System=AppDES  NodeID=1  DestinationNode=1  ApplicationState=0  TTL=127  SourceRate=1  TotalPackets=1  SimulateUsing=Code generation
      mask Type: AppDES
      mask Display:
      | disp('AppDES');
      | port_label('input',1,'transportPDUIn');
      | port_label('output',1,'transportPDUOut');
      | port_label('output',2,'networkConfig');
  BLE channel : BLEMeshLib/BLE Channel  RangePropagationLoss=On  FSPLModel=On  RxRange=8  NodePosition=NodePosition  NodeID=NodeID  SimulateUsing=Code generation
  Entity Multicast : EntityMulticast  InputPortMessageModes=m  MulticastTag=channel
  Entity Replicator : EntityReplicator  InputPortMessageModes=m  OutputPortMessageModes=m,m
  Link layer : BLEMeshLib/Link layer  RandomAdvertising=On  AdvertisingInterval=20  ScanInterval=30  NodeID=NodeID  SimulateUsing=Code generation  mask(helperBLEMeshLinkLayerDES){}
  Multicast Receive Queue : Queue  OutputPortMessageModes=m  EntityArrivalSource=Multicast  MulticastTag=channel
  Network layer : BLEMeshLib/Network layer  Relay=Off  ElementAddresses=ElementAddress  NetworkTransmitCount=3  NetworkTransmitInterval=30  RelayRetransmitCount=3  RelayRetransmitInterval=30  NodeID=NodeID  SimulateUsing=Code generation
  PHY Rx : BLEMeshLib/PHY Rx  NoiseFigure=0  NodeID=NodeID  SimulateUsing=Interpreted execution
  PHY Tx : BLEMeshLib/PHY Tx  TxPower=0  NodePosition=NodePosition  NodeID=NodeID  SimulateUsing=Interpreted execution
  wires:
  Link layer/4 -> [LLReqToPHYRx]
  Link layer/2 -> [PDUToPHY]
  Link layer/3 -> [LLReqToPHYTx]
  Link layer/1 -> [PDUFromLinkLayer]
  [PDUToNetworkLayer] -> Network layer/1
  Network layer/1 -> [PDUToApplication]
  [PDUFromLinkLayer] -> Network layer/2
  Entity Replicator/1 -> PHY Rx/1
  PHY Rx/1 -> [PDUFromPHY]
  BLE channel/1 -> PHY Rx/2
  PHY Tx/1 -> Entity Multicast/1
  [LLReqToPHYRx] -> Entity Replicator/1
  Multicast Receive Queue/1 -> BLE channel/2
  Entity Replicator/2 -> BLE channel/1
  [LLReqToPHYTx] -> PHY Tx/1
  [PDUToPHY] -> PHY Tx/2
  Network layer/2 -> [PDUToLinkLayer]
  [PDUToLinkLayer] -> Link layer/1
  [PDUFromPHY] -> Link layer/2
  AppDES/1 -> [PDUToNetworkLayer]
  [PDUToApplication] -> AppDES/1
  [NetworkConfig] -> Network layer/3
  AppDES/2 -> [NetworkConfig]

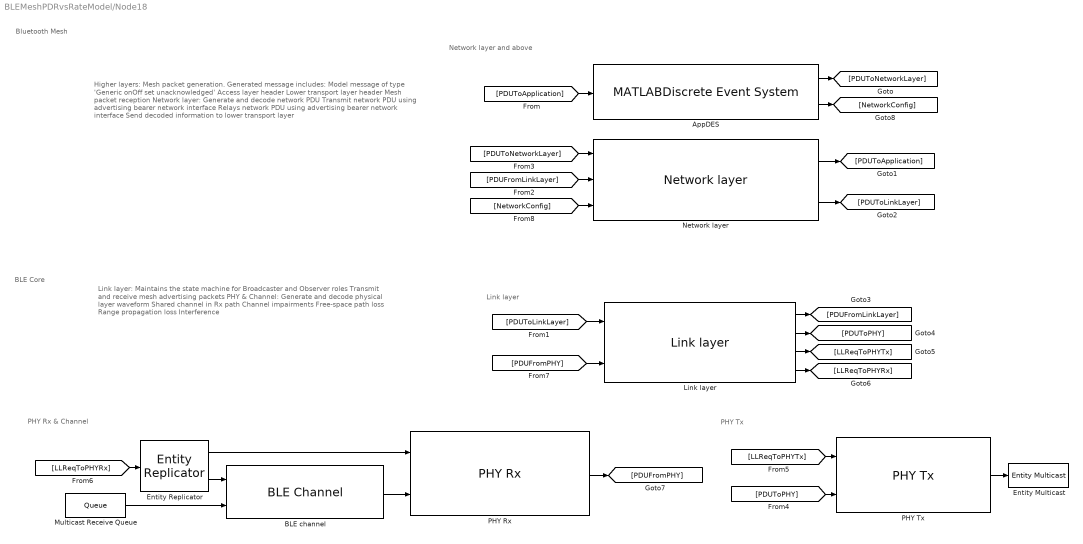
== system BLEMeshPDRvsRateModel/Node18 ==
  note: Network layer and above
  note: Link layer
  note: Link layer:
      | Maintains the state machine for Broadcaster and Observer roles
      | Transmit and receive mesh advertising packets
      |
      | PHY & Channel:
      | Generate and decode physical layer waveform
      | Shared channel in Rx path
      | Channel impairments
      | Free-space path loss
      | Range propagation loss
      | Interference
  note: BLE Core
  note: Bluetooth Mesh
  note: PHY Rx & Channel
  note: PHY Tx
  note: Higher layers:
      | Mesh packet generation. Generated message includes:
      | Model message of type 'Generic onOff set unacknowledged'
      | Access layer header
      | Lower transport layer header
      | Mesh packet reception
      |
      | Network layer:
      | Generate and decode network PDU
      | Transmit network PDU using advertising bearer network interface
      | Relays network PDU using advertising bearer network interface
      | Send decoded information to lower transport layer
  AppDES : MATLABDiscreteEventSystem  InputPortMessageModes=m  OutputPortMessageModes=m,m  System=AppDES  NodeID=1  DestinationNode=1  ApplicationState=0  TTL=127  SourceRate=1  TotalPackets=1  SimulateUsing=Code generation
      mask Type: AppDES
      mask Display:
      | disp('AppDES');
      | port_label('input',1,'transportPDUIn');
      | port_label('output',1,'transportPDUOut');
      | port_label('output',2,'networkConfig');
  BLE channel : BLEMeshLib/BLE Channel  RangePropagationLoss=On  FSPLModel=On  RxRange=8  NodePosition=NodePosition  NodeID=NodeID  SimulateUsing=Code generation
  Entity Multicast : EntityMulticast  InputPortMessageModes=m  MulticastTag=channel
  Entity Replicator : EntityReplicator  InputPortMessageModes=m  OutputPortMessageModes=m,m
  Link layer : BLEMeshLib/Link layer  RandomAdvertising=On  AdvertisingInterval=20  ScanInterval=30  NodeID=NodeID  SimulateUsing=Code generation  mask(helperBLEMeshLinkLayerDES){}
  Multicast Receive Queue : Queue  OutputPortMessageModes=m  EntityArrivalSource=Multicast  MulticastTag=channel
  Network layer : BLEMeshLib/Network layer  Relay=Off  ElementAddresses=ElementAddress  NetworkTransmitCount=3  NetworkTransmitInterval=30  RelayRetransmitCount=3  RelayRetransmitInterval=30  NodeID=NodeID  SimulateUsing=Code generation
  PHY Rx : BLEMeshLib/PHY Rx  NoiseFigure=0  NodeID=NodeID  SimulateUsing=Interpreted execution
  PHY Tx : BLEMeshLib/PHY Tx  TxPower=0  NodePosition=NodePosition  NodeID=NodeID  SimulateUsing=Interpreted execution
  wires:
  Link layer/4 -> [LLReqToPHYRx]
  Link layer/2 -> [PDUToPHY]
  Link layer/3 -> [LLReqToPHYTx]
  Link layer/1 -> [PDUFromLinkLayer]
  [PDUToNetworkLayer] -> Network layer/1
  Network layer/1 -> [PDUToApplication]
  [PDUFromLinkLayer] -> Network layer/2
  Entity Replicator/1 -> PHY Rx/1
  PHY Rx/1 -> [PDUFromPHY]
  BLE channel/1 -> PHY Rx/2
  PHY Tx/1 -> Entity Multicast/1
  [LLReqToPHYRx] -> Entity Replicator/1
  Multicast Receive Queue/1 -> BLE channel/2
  Entity Replicator/2 -> BLE channel/1
  [LLReqToPHYTx] -> PHY Tx/1
  [PDUToPHY] -> PHY Tx/2
  Network layer/2 -> [PDUToLinkLayer]
  [PDUToLinkLayer] -> Link layer/1
  [PDUFromPHY] -> Link layer/2
  AppDES/1 -> [PDUToNetworkLayer]
  [PDUToApplication] -> AppDES/1
  [NetworkConfig] -> Network layer/3
  AppDES/2 -> [NetworkConfig]

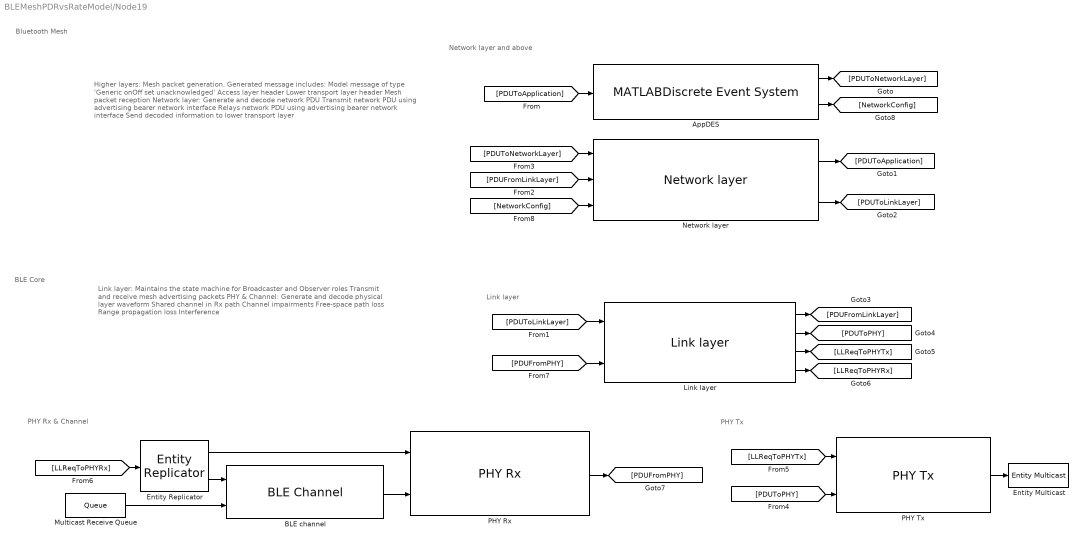
== system BLEMeshPDRvsRateModel/Node19 ==
  note: Network layer and above
  note: Link layer
  note: Link layer:
      | Maintains the state machine for Broadcaster and Observer roles
      | Transmit and receive mesh advertising packets
      |
      | PHY & Channel:
      | Generate and decode physical layer waveform
      | Shared channel in Rx path
      | Channel impairments
      | Free-space path loss
      | Range propagation loss
      | Interference
  note: BLE Core
  note: Bluetooth Mesh
  note: PHY Rx & Channel
  note: PHY Tx
  note: Higher layers:
      | Mesh packet generation. Generated message includes:
      | Model message of type 'Generic onOff set unacknowledged'
      | Access layer header
      | Lower transport layer header
      | Mesh packet reception
      |
      | Network layer:
      | Generate and decode network PDU
      | Transmit network PDU using advertising bearer network interface
      | Relays network PDU using advertising bearer network interface
      | Send decoded information to lower transport layer
  AppDES : MATLABDiscreteEventSystem  InputPortMessageModes=m  OutputPortMessageModes=m,m  System=AppDES  NodeID=1  DestinationNode=1  ApplicationState=0  TTL=127  SourceRate=1  TotalPackets=1  SimulateUsing=Code generation
      mask Type: AppDES
      mask Display:
      | disp('AppDES');
      | port_label('input',1,'transportPDUIn');
      | port_label('output',1,'transportPDUOut');
      | port_label('output',2,'networkConfig');
  BLE channel : BLEMeshLib/BLE Channel  RangePropagationLoss=On  FSPLModel=On  RxRange=8  NodePosition=NodePosition  NodeID=NodeID  SimulateUsing=Code generation
  Entity Multicast : EntityMulticast  InputPortMessageModes=m  MulticastTag=channel
  Entity Replicator : EntityReplicator  InputPortMessageModes=m  OutputPortMessageModes=m,m
  Link layer : BLEMeshLib/Link layer  RandomAdvertising=On  AdvertisingInterval=20  ScanInterval=30  NodeID=NodeID  SimulateUsing=Code generation  mask(helperBLEMeshLinkLayerDES){}
  Multicast Receive Queue : Queue  OutputPortMessageModes=m  EntityArrivalSource=Multicast  MulticastTag=channel
  Network layer : BLEMeshLib/Network layer  Relay=On  ElementAddresses=ElementAddress  NetworkTransmitCount=3  NetworkTransmitInterval=30  RelayRetransmitCount=3  RelayRetransmitInterval=30  NodeID=NodeID  SimulateUsing=Code generation
  PHY Rx : BLEMeshLib/PHY Rx  NoiseFigure=0  NodeID=NodeID  SimulateUsing=Interpreted execution
  PHY Tx : BLEMeshLib/PHY Tx  TxPower=0  NodePosition=NodePosition  NodeID=NodeID  SimulateUsing=Interpreted execution
  wires:
  Link layer/4 -> [LLReqToPHYRx]
  Link layer/2 -> [PDUToPHY]
  Link layer/3 -> [LLReqToPHYTx]
  Link layer/1 -> [PDUFromLinkLayer]
  [PDUToNetworkLayer] -> Network layer/1
  Network layer/1 -> [PDUToApplication]
  [PDUFromLinkLayer] -> Network layer/2
  Entity Replicator/1 -> PHY Rx/1
  PHY Rx/1 -> [PDUFromPHY]
  BLE channel/1 -> PHY Rx/2
  PHY Tx/1 -> Entity Multicast/1
  [LLReqToPHYRx] -> Entity Replicator/1
  Multicast Receive Queue/1 -> BLE channel/2
  Entity Replicator/2 -> BLE channel/1
  [LLReqToPHYTx] -> PHY Tx/1
  [PDUToPHY] -> PHY Tx/2
  Network layer/2 -> [PDUToLinkLayer]
  [PDUToLinkLayer] -> Link layer/1
  [PDUFromPHY] -> Link layer/2
  AppDES/1 -> [PDUToNetworkLayer]
  [PDUToApplication] -> AppDES/1
  [NetworkConfig] -> Network layer/3
  AppDES/2 -> [NetworkConfig]

== system BLEMeshPDRvsRateModel/Node2 ==
  note: Network layer and above
  note: Link layer
  note: Link layer:
      | Maintains the state machine for Broadcaster and Observer roles
      | Transmit and receive mesh advertising packets
      |
      | PHY & Channel:
      | Generate and decode physical layer waveform
      | Shared channel in Rx path
      | Channel impairments
      | Free-space path loss
      | Range propagation loss
      | Interference
  note: BLE Core
  note: Bluetooth Mesh
  note: PHY Rx & Channel
  note: PHY Tx
  note: Higher layers:
      | Mesh packet generation. Generated message includes:
      | Model message of type 'Generic onOff set unacknowledged'
      | Access layer header
      | Lower transport layer header
      | Mesh packet reception
      |
      | Network layer:
      | Generate and decode network PDU
      | Transmit network PDU using advertising bearer network interface
      | Relays network PDU using advertising bearer network interface
      | Send decoded information to lower transport layer
  AppDES : MATLABDiscreteEventSystem  InputPortMessageModes=m  OutputPortMessageModes=m,m  System=AppDES  NodeID=1  DestinationNode=1  ApplicationState=0  TTL=127  SourceRate=1  TotalPackets=1  SimulateUsing=Code generation
      mask Type: AppDES
      mask Display:
      | disp('AppDES');
      | port_label('input',1,'transportPDUIn');
      | port_label('output',1,'transportPDUOut');
      | port_label('output',2,'networkConfig');
  BLE channel : BLEMeshLib/BLE Channel  RangePropagationLoss=On  FSPLModel=On  RxRange=8  NodePosition=NodePosition  NodeID=NodeID  SimulateUsing=Code generation
  Entity Multicast : EntityMulticast  InputPortMessageModes=m  MulticastTag=channel
  Entity Replicator : EntityReplicator  InputPortMessageModes=m  OutputPortMessageModes=m,m
  Link layer : BLEMeshLib/Link layer  RandomAdvertising=On  AdvertisingInterval=20  ScanInterval=30  NodeID=NodeID  SimulateUsing=Code generation  mask(helperBLEMeshLinkLayerDES){}
  Multicast Receive Queue : Queue  OutputPortMessageModes=m  EntityArrivalSource=Multicast  MulticastTag=channel
  Network layer : BLEMeshLib/Network layer  Relay=On  ElementAddresses=ElementAddress  NetworkTransmitCount=3  NetworkTransmitInterval=30  RelayRetransmitCount=3  RelayRetransmitInterval=30  NodeID=NodeID  SimulateUsing=Code generation
  PHY Rx : BLEMeshLib/PHY Rx  NoiseFigure=0  NodeID=NodeID  SimulateUsing=Interpreted execution
  PHY Tx : BLEMeshLib/PHY Tx  TxPower=0  NodePosition=NodePosition  NodeID=NodeID  SimulateUsing=Interpreted execution
  wires:
  Link layer/4 -> [LLReqToPHYRx]
  Link layer/2 -> [PDUToPHY]
  Link layer/3 -> [LLReqToPHYTx]
  Link layer/1 -> [PDUFromLinkLayer]
  [PDUToNetworkLayer] -> Network layer/1
  Network layer/1 -> [PDUToApplication]
  [PDUFromLinkLayer] -> Network layer/2
  Entity Replicator/1 -> PHY Rx/1
  PHY Rx/1 -> [PDUFromPHY]
  BLE channel/1 -> PHY Rx/2
  PHY Tx/1 -> Entity Multicast/1
  [LLReqToPHYRx] -> Entity Replicator/1
  Multicast Receive Queue/1 -> BLE channel/2
  Entity Replicator/2 -> BLE channel/1
  [LLReqToPHYTx] -> PHY Tx/1
  [PDUToPHY] -> PHY Tx/2
  Network layer/2 -> [PDUToLinkLayer]
  [PDUToLinkLayer] -> Link layer/1
  [PDUFromPHY] -> Link layer/2
  AppDES/1 -> [PDUToNetworkLayer]
  [PDUToApplication] -> AppDES/1
  [NetworkConfig] -> Network layer/3
  AppDES/2 -> [NetworkConfig]

== system BLEMeshPDRvsRateModel/Node20 ==
  note: Network layer and above
  note: Link layer
  note: Link layer:
      | Maintains the state machine for Broadcaster and Observer roles
      | Transmit and receive mesh advertising packets
      |
      | PHY & Channel:
      | Generate and decode physical layer waveform
      | Shared channel in Rx path
      | Channel impairments
      | Free-space path loss
      | Range propagation loss
      | Interference
  note: BLE Core
  note: Bluetooth Mesh
  note: PHY Rx & Channel
  note: PHY Tx
  note: Higher layers:
      | Mesh packet generation. Generated message includes:
      | Model message of type 'Generic onOff set unacknowledged'
      | Access layer header
      | Lower transport layer header
      | Mesh packet reception
      |
      | Network layer:
      | Generate and decode network PDU
      | Transmit network PDU using advertising bearer network interface
      | Relays network PDU using advertising bearer network interface
      | Send decoded information to lower transport layer
  AppDES : MATLABDiscreteEventSystem  InputPortMessageModes=m  OutputPortMessageModes=m,m  System=AppDES  NodeID=1  DestinationNode=1  ApplicationState=0  TTL=127  SourceRate=1  TotalPackets=1  SimulateUsing=Code generation
      mask Type: AppDES
      mask Display:
      | disp('AppDES');
      | port_label('input',1,'transportPDUIn');
      | port_label('output',1,'transportPDUOut');
      | port_label('output',2,'networkConfig');
  BLE channel : BLEMeshLib/BLE Channel  RangePropagationLoss=On  FSPLModel=On  RxRange=8  NodePosition=NodePosition  NodeID=NodeID  SimulateUsing=Code generation
  Entity Multicast : EntityMulticast  InputPortMessageModes=m  MulticastTag=channel
  Entity Replicator : EntityReplicator  InputPortMessageModes=m  OutputPortMessageModes=m,m
  Link layer : BLEMeshLib/Link layer  RandomAdvertising=On  AdvertisingInterval=20  ScanInterval=30  NodeID=NodeID  SimulateUsing=Code generation  mask(helperBLEMeshLinkLayerDES){}
  Multicast Receive Queue : Queue  OutputPortMessageModes=m  EntityArrivalSource=Multicast  MulticastTag=channel
  Network layer : BLEMeshLib/Network layer  Relay=On  ElementAddresses=ElementAddress  NetworkTransmitCount=3  NetworkTransmitInterval=30  RelayRetransmitCount=3  RelayRetransmitInterval=30  NodeID=NodeID  SimulateUsing=Code generation
  PHY Rx : BLEMeshLib/PHY Rx  NoiseFigure=0  NodeID=NodeID  SimulateUsing=Interpreted execution
  PHY Tx : BLEMeshLib/PHY Tx  TxPower=0  NodePosition=NodePosition  NodeID=NodeID  SimulateUsing=Interpreted execution
  wires:
  Link layer/4 -> [LLReqToPHYRx]
  Link layer/2 -> [PDUToPHY]
  Link layer/3 -> [LLReqToPHYTx]
  Link layer/1 -> [PDUFromLinkLayer]
  [PDUToNetworkLayer] -> Network layer/1
  Network layer/1 -> [PDUToApplication]
  [PDUFromLinkLayer] -> Network layer/2
  Entity Replicator/1 -> PHY Rx/1
  PHY Rx/1 -> [PDUFromPHY]
  BLE channel/1 -> PHY Rx/2
  PHY Tx/1 -> Entity Multicast/1
  [LLReqToPHYRx] -> Entity Replicator/1
  Multicast Receive Queue/1 -> BLE channel/2
  Entity Replicator/2 -> BLE channel/1
  [LLReqToPHYTx] -> PHY Tx/1
  [PDUToPHY] -> PHY Tx/2
  Network layer/2 -> [PDUToLinkLayer]
  [PDUToLinkLayer] -> Link layer/1
  [PDUFromPHY] -> Link layer/2
  AppDES/1 -> [PDUToNetworkLayer]
  [PDUToApplication] -> AppDES/1
  [NetworkConfig] -> Network layer/3
  AppDES/2 -> [NetworkConfig]

== system BLEMeshPDRvsRateModel/Node21 ==
  note: Network layer and above
  note: Link layer
  note: Link layer:
      | Maintains the state machine for Broadcaster and Observer roles
      | Transmit and receive mesh advertising packets
      |
      | PHY & Channel:
      | Generate and decode physical layer waveform
      | Shared channel in Rx path
      | Channel impairments
      | Free-space path loss
      | Range propagation loss
      | Interference
  note: BLE Core
  note: Bluetooth Mesh
  note: PHY Rx & Channel
  note: PHY Tx
  note: Higher layers:
      | Mesh packet generation. Generated message includes:
      | Model message of type 'Generic onOff set unacknowledged'
      | Access layer header
      | Lower transport layer header
      | Mesh packet reception
      |
      | Network layer:
      | Generate and decode network PDU
      | Transmit network PDU using advertising bearer network interface
      | Relays network PDU using advertising bearer network interface
      | Send decoded information to lower transport layer
  AppDES : MATLABDiscreteEventSystem  InputPortMessageModes=m  OutputPortMessageModes=m,m  System=AppDES  NodeID=1  DestinationNode=1  ApplicationState=0  TTL=127  SourceRate=1  TotalPackets=1  SimulateUsing=Code generation
      mask Type: AppDES
      mask Display:
      | disp('AppDES');
      | port_label('input',1,'transportPDUIn');
      | port_label('output',1,'transportPDUOut');
      | port_label('output',2,'networkConfig');
  BLE channel : BLEMeshLib/BLE Channel  RangePropagationLoss=On  FSPLModel=On  RxRange=8  NodePosition=NodePosition  NodeID=NodeID  SimulateUsing=Code generation
  Entity Multicast : EntityMulticast  InputPortMessageModes=m  MulticastTag=channel
  Entity Replicator : EntityReplicator  InputPortMessageModes=m  OutputPortMessageModes=m,m
  Link layer : BLEMeshLib/Link layer  RandomAdvertising=On  AdvertisingInterval=20  ScanInterval=30  NodeID=NodeID  SimulateUsing=Code generation  mask(helperBLEMeshLinkLayerDES){}
  Multicast Receive Queue : Queue  OutputPortMessageModes=m  EntityArrivalSource=Multicast  MulticastTag=channel
  Network layer : BLEMeshLib/Network layer  Relay=On  ElementAddresses=ElementAddress  NetworkTransmitCount=3  NetworkTransmitInterval=30  RelayRetransmitCount=3  RelayRetransmitInterval=30  NodeID=NodeID  SimulateUsing=Code generation
  PHY Rx : BLEMeshLib/PHY Rx  NoiseFigure=0  NodeID=NodeID  SimulateUsing=Interpreted execution
  PHY Tx : BLEMeshLib/PHY Tx  TxPower=0  NodePosition=NodePosition  NodeID=NodeID  SimulateUsing=Interpreted execution
  wires:
  Link layer/4 -> [LLReqToPHYRx]
  Link layer/2 -> [PDUToPHY]
  Link layer/3 -> [LLReqToPHYTx]
  Link layer/1 -> [PDUFromLinkLayer]
  [PDUToNetworkLayer] -> Network layer/1
  Network layer/1 -> [PDUToApplication]
  [PDUFromLinkLayer] -> Network layer/2
  Entity Replicator/1 -> PHY Rx/1
  PHY Rx/1 -> [PDUFromPHY]
  BLE channel/1 -> PHY Rx/2
  PHY Tx/1 -> Entity Multicast/1
  [LLReqToPHYRx] -> Entity Replicator/1
  Multicast Receive Queue/1 -> BLE channel/2
  Entity Replicator/2 -> BLE channel/1
  [LLReqToPHYTx] -> PHY Tx/1
  [PDUToPHY] -> PHY Tx/2
  Network layer/2 -> [PDUToLinkLayer]
  [PDUToLinkLayer] -> Link layer/1
  [PDUFromPHY] -> Link layer/2
  AppDES/1 -> [PDUToNetworkLayer]
  [PDUToApplication] -> AppDES/1
  [NetworkConfig] -> Network layer/3
  AppDES/2 -> [NetworkConfig]

== system BLEMeshPDRvsRateModel/Node22 ==
  note: Network layer and above
  note: Link layer
  note: Link layer:
      | Maintains the state machine for Broadcaster and Observer roles
      | Transmit and receive mesh advertising packets
      |
      | PHY & Channel:
      | Generate and decode physical layer waveform
      | Shared channel in Rx path
      | Channel impairments
      | Free-space path loss
      | Range propagation loss
      | Interference
  note: BLE Core
  note: Bluetooth Mesh
  note: PHY Rx & Channel
  note: PHY Tx
  note: Higher layers:
      | Mesh packet generation. Generated message includes:
      | Model message of type 'Generic onOff set unacknowledged'
      | Access layer header
      | Lower transport layer header
      | Mesh packet reception
      |
      | Network layer:
      | Generate and decode network PDU
      | Transmit network PDU using advertising bearer network interface
      | Relays network PDU using advertising bearer network interface
      | Send decoded information to lower transport layer
  AppDES : MATLABDiscreteEventSystem  InputPortMessageModes=m  OutputPortMessageModes=m,m  System=AppDES  NodeID=1  DestinationNode=1  ApplicationState=0  TTL=127  SourceRate=1  TotalPackets=1  SimulateUsing=Code generation
      mask Type: AppDES
      mask Display:
      | disp('AppDES');
      | port_label('input',1,'transportPDUIn');
      | port_label('output',1,'transportPDUOut');
      | port_label('output',2,'networkConfig');
  BLE channel : BLEMeshLib/BLE Channel  RangePropagationLoss=On  FSPLModel=On  RxRange=8  NodePosition=NodePosition  NodeID=NodeID  SimulateUsing=Code generation
  Entity Multicast : EntityMulticast  InputPortMessageModes=m  MulticastTag=channel
  Entity Replicator : EntityReplicator  InputPortMessageModes=m  OutputPortMessageModes=m,m
  Link layer : BLEMeshLib/Link layer  RandomAdvertising=On  AdvertisingInterval=20  ScanInterval=30  NodeID=NodeID  SimulateUsing=Code generation  mask(helperBLEMeshLinkLayerDES){}
  Multicast Receive Queue : Queue  OutputPortMessageModes=m  EntityArrivalSource=Multicast  MulticastTag=channel
  Network layer : BLEMeshLib/Network layer  Relay=On  ElementAddresses=ElementAddress  NetworkTransmitCount=3  NetworkTransmitInterval=30  RelayRetransmitCount=3  RelayRetransmitInterval=30  NodeID=NodeID  SimulateUsing=Code generation
  PHY Rx : BLEMeshLib/PHY Rx  NoiseFigure=0  NodeID=NodeID  SimulateUsing=Interpreted execution
  PHY Tx : BLEMeshLib/PHY Tx  TxPower=0  NodePosition=NodePosition  NodeID=NodeID  SimulateUsing=Interpreted execution
  wires:
  Link layer/4 -> [LLReqToPHYRx]
  Link layer/2 -> [PDUToPHY]
  Link layer/3 -> [LLReqToPHYTx]
  Link layer/1 -> [PDUFromLinkLayer]
  [PDUToNetworkLayer] -> Network layer/1
  Network layer/1 -> [PDUToApplication]
  [PDUFromLinkLayer] -> Network layer/2
  Entity Replicator/1 -> PHY Rx/1
  PHY Rx/1 -> [PDUFromPHY]
  BLE channel/1 -> PHY Rx/2
  PHY Tx/1 -> Entity Multicast/1
  [LLReqToPHYRx] -> Entity Replicator/1
  Multicast Receive Queue/1 -> BLE channel/2
  Entity Replicator/2 -> BLE channel/1
  [LLReqToPHYTx] -> PHY Tx/1
  [PDUToPHY] -> PHY Tx/2
  Network layer/2 -> [PDUToLinkLayer]
  [PDUToLinkLayer] -> Link layer/1
  [PDUFromPHY] -> Link layer/2
  AppDES/1 -> [PDUToNetworkLayer]
  [PDUToApplication] -> AppDES/1
  [NetworkConfig] -> Network layer/3
  AppDES/2 -> [NetworkConfig]
